simulink library "fzgbib"  (Simulink 4.1.1)
values from neighbouring files (symbols this model uses):
  a_Fzg_max = 2    [PedalInterp_para.m]
  a_Fzg_min = -2    [PedalInterp_para.m]
  gang0 = 1    [PedalInterp_para.m]
  gang_vec = [1 2 3 4]    [PedalInterp_para.m]
  lambda_gang = [1.3 1.25  1.17  1.05]    [PedalInterp_para.m]
  M_Br_max = 4000    [PedalInterp_para.m]
undefined symbols (not defined in the file or in its folder): A, cw, gang, i_d, i_g, m_ab_100pro, m_ab_70pro, m_Fzg, M_mot_max, M_mot_min, n_mot0, n_mot_max, n_mot_min, p_anteil, r_dyn, rho, t_sch, v_bereich, v_Fzg_ms0
libraries: simulink3 x1
(part 2 of 2)

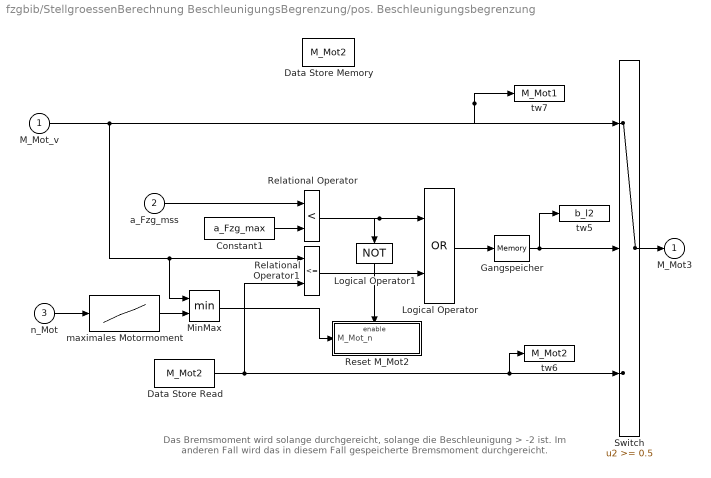
== system fzgbib/StellgroessenBerechnung BeschleunigungsBegrenzung/pos. Beschleunigungsbegrenzung ==
  note: Das Bremsmoment wird solange durchgereicht, solange die Beschleunigung > -2 ist.
      | Im anderen Fall wird das in diesem Fall gespeicherte Bremsmoment durchgereicht.
  M_Mot_v : Inport  Port=1  LatchInput=off
  a_Fzg_mss : Inport  Port=2  LatchInput=off
  "n_Mot " : Inport  Port=3  LatchInput=off
  Constant1 : Constant  Value=a_Fzg_max
  Data Store Memory : DataStoreMemory  DataStoreName=M_Mot2  InitialValue=0
  Data Store Read : DataStoreRead  DataStoreName=M_Mot2  SampleTime=-1
  Gangspeicher : Memory  X0=1  InheritSampleTime=off
      settings: RTWStateStorageClass=Auto
  Logical Operator : Logic  Operator=OR  Inputs=2
  Logical Operator1 : Logic  Orientation=down  Operator=NOT  Inputs=1
  MinMax : MinMax  Function=min  Inputs=2
  Relational Operator : RelationalOperator  Operator=<
  Relational Operator1 : RelationalOperator  Operator=<=
  Reset M_Mot2 : Subsystem  TreatAsAtomicUnit=on
      settings: RTWFcnNameOpts=Auto  RTWFileNameOpts=Auto
  Switch : Switch  Threshold=0.5
  maximales Motormoment : Lookup  InputValues=[0 n_mot_max]  OutputValues=[M_mot_max(1) M_mot_max]
  tw5 : ToWorkspace  VariableName=b_l2  SampleTime=0  SaveFormat=Array
      settings: MaxDataPoints=speicher
  tw6 : ToWorkspace  VariableName=M_Mot2  SampleTime=0  SaveFormat=Array
      settings: MaxDataPoints=speicher
  tw7 : ToWorkspace  VariableName=M_Mot1  SampleTime=0  SaveFormat=Array
      settings: MaxDataPoints=speicher
  M_Mot3 : Outport  Port=1  InitialOutput=0
  wires:
  maximales Motormoment/1 -> MinMax/2
  "n_Mot "/1 -> maximales Motormoment/1
  MinMax/1 -> Reset M_Mot2/1(M_Mot_n)
  a_Fzg_mss/1 -> Relational Operator/1
  Logical Operator1/1 -> Reset M_Mot2/Enable
  Relational Operator/1 -> Logical Operator1/1, Logical Operator/1
  M_Mot_v/1 -> MinMax/1, Relational Operator1/1, tw7/1, Switch/1
  Gangspeicher/1 -> tw5/1, Switch/2
  Logical Operator/1 -> Gangspeicher/1
  Data Store Read/1 -> Relational Operator1/2, tw6/1, Switch/3
  Relational Operator1/1 -> Logical Operator/2
  Constant1/1 -> Relational Operator/2
  Switch/1 -> M_Mot3/1

== system fzgbib/Watchdog 1/error dedected ==
  Enable : EnablePort
  Constant : Constant  Value=1
  max_overshoot_flag [0/1] : Outport  Port=1  InitialOutput=0
  wires:
  Constant/1 -> max_overshoot_flag [0/1]/1

== system fzgbib/Watchdog 1/save actual and reference speed ==
  "actual  speed " : Inport  Port=1  LatchInput=off
  "reference  speed  " : Inport  Port=2  LatchInput=off
  Enable : EnablePort
  actual  speed hold : Outport  Port=1  InitialOutput=0
  reference  speed hold : Outport  Port=2  InitialOutput=0
  wires:
  "reference  speed  "/1 -> reference  speed hold/1
  "actual  speed "/1 -> actual  speed hold/1

== system fzgbib/Watchdog 2/error dedected ==
  Enable : EnablePort
  Constant : Constant  Value=1
  step_response_flag [0/1] : Outport  Port=1  InitialOutput=0
  wires:
  Constant/1 -> step_response_flag [0/1]/1

== system fzgbib/Watchdog 2/save actual time and reference speed ==
  "actual time " : Inport  Port=1  LatchInput=off
  "reference speed  " : Inport  Port=2  LatchInput=off
  Enable : EnablePort
  actual time hold : Outport  Port=1  InitialOutput=0
  reference speed hold : Outport  Port=2  InitialOutput=0
  wires:
  "reference speed  "/1 -> reference speed hold/1
  "actual time "/1 -> actual time hold/1

== system fzgbib/Fahrzeugmodell/Fahrwiderstaende/Schaltdauer ==
  note: Eine Wunschgangaenderung wird registriert und der neue Wunschgang solange im Speicher abgelegt,
      | bis die Schlatung beendet ist.
  note: 14.5.1996 Dieter Hoetzer / letzte aenderung
  Gang_w : Inport  Port=1  LatchInput=off
  Memory1 : Memory  X0=1  InheritSampleTime=off
      settings: RTWStateStorageClass=Auto
  Relational Operator1 : RelationalOperator  Operator=~=
  Schaltdauer : TransportDelay  DelayTime=t_sch  InitialInput=1  BufferSize=1024  PadeOrder=0
  Speicher : Memory  X0=1  InheritSampleTime=off
      settings: RTWStateStorageClass=Auto
  Switch : Switch  Threshold=0.5
  ungleich : RelationalOperator  Operator=~=
  k_l : Outport  Port=1  InitialOutput=0
  wires:
  Switch/1 -> Speicher/1
  Gang_w/1 -> ungleich/1, Switch/1, Memory1/1
  Memory1/1 -> ungleich/2
  ungleich/1 -> Switch/2
  Speicher/1 -> Switch/3, Relational Operator1/1, Schaltdauer/1
  Schaltdauer/1 -> Relational Operator1/2
  Relational Operator1/1 -> k_l/1

== system fzgbib/Fahrzeugmodell/Fahrzeugdynamik/Band-Limited White Noise ==
  Gain : Gain  Gain=[sqrt(Cov)]/[sqrt(Ts)]  Multiplication=Element-wise(K.*u)  SaturateOnIntegerOverflow=on
  White Noise : RandomNumber  Mean=0  Variance=1  Seed=seed  SampleTime=-1
  Zero-Order Hold : ZeroOrderHold  SampleTime=Ts
  Out_1 : Outport  Port=1  InitialOutput=0
  wires:
  Zero-Order Hold/1 -> Gain/1
  Gain/1 -> Out_1/1
  White Noise/1 -> Zero-Order Hold/1

== system fzgbib/Gangberechnung/Hoch-Rueckschaltung Auswahl/Halte Zeit ==
  Clock : Inport  Port=1  LatchInput=off
  Enable : EnablePort
  Write : DataStoreWrite  DataStoreName=time1  SampleTime=-1
  wires:
  Clock/1 -> Write/1

== system fzgbib/GeschwindigkeitsRegelung/Stoergroessenkompensation/Luft- und Rollwiderstand ==
  note: Keine Steigung beruecksichtigt
  v_Fzg : Inport  Port=1  LatchInput=off
  F_L Berechnung : Fcn  Expr=u*rho*A/2*cw
  F_R Berechnung : Fcn  Expr=(u>0.1)*f_r*m_Fzg*g
  Fcn : Fcn  Expr=u*r_dyn
  Product : Product  Inputs=2  Multiplication=Element-wise(.*)  SaturateOnIntegerOverflow=on
  Sum : Sum  Inputs=++  SaturateOnIntegerOverflow=on
  M_G : Outport  Port=1  InitialOutput=0
  wires:
  Fcn/1 -> M_G/1
  Sum/1 -> Fcn/1
  F_L Berechnung/1 -> Sum/1
  F_R Berechnung/1 -> Sum/2
  v_Fzg/1 -> F_R Berechnung/1, Product/1, Product/2
  Product/1 -> F_L Berechnung/1

== system fzgbib/GeschwindigkeitsRegelung/Stoergroessenkompensation/Sollverhalten Fahrzeug mit P-Regler1 ==
  v_soll : Inport  Port=1  LatchInput=off
  v_Fzg : Inport  Port=2  LatchInput=off
  GR_aktiv_l : Inport  Port=3  LatchInput=off
  1/T : Fcn  Expr=1/u
  Grenze3 : Constant  Value=r_dyn*m_Fzg/p_anteil
  Grenze4 : Constant  Value=0.1
  Integrator : Integrator  ExternalReset=none  InitialConditionSource=internal  InitialCondition=v_Fzg_ms0  LimitOutput=off  UpperSaturationLimit=inf  LowerSaturationLimit=-inf  ShowSaturationPort=off  ShowStatePort=off  AbsoluteTolerance=auto
  Product : Product  Inputs=2  Multiplication=Element-wise(.*)  SaturateOnIntegerOverflow=on
  Reglerabweichung : Sum  Inputs=-+  SaturateOnIntegerOverflow=on
  Switch : Switch  Threshold=0.5
  Switch1 : Switch  Threshold=0.5
  v_Fzg1 : Outport  Port=1  InitialOutput=0
  wires:
  Integrator/1 -> v_Fzg1/1, Reglerabweichung/1
  Product/1 -> Integrator/1
  Switch/1 -> 1/T/1
  Reglerabweichung/1 -> Product/1
  1/T/1 -> Product/2
  Grenze4/1 -> Switch/3
  Grenze3/1 -> Switch/1
  Switch1/1 -> Reglerabweichung/2
  v_soll/1 -> Switch1/1
  v_Fzg/1 -> Switch1/3
  GR_aktiv_l/1 -> Switch/2, Switch1/2

== system fzgbib/StellgroessenBerechnung BeschleunigungsBegrenzung/neg. Beschleunigungsbegrenzung/Reset M_Br2 ==
  M_Br_n : Inport  Port=1  LatchInput=off
  a_Fzg_mss : Inport  Port=2  LatchInput=off
  Enable : EnablePort
  Constant1 : Constant  Value=a_Fzg_min
  Constant2 : Constant  Value=10
  Data Store Write : DataStoreWrite  DataStoreName=M_Br2  SampleTime=-1
  Product : Product  Inputs=2  Multiplication=Element-wise(.*)  SaturateOnIntegerOverflow=on
  Sum : Sum  Inputs=++  SaturateOnIntegerOverflow=on
  Sum1 : Sum  Inputs=+-  SaturateOnIntegerOverflow=on
  wires:
  Constant2/1 -> Product/1
  Constant1/1 -> Sum1/2
  a_Fzg_mss/1 -> Sum1/1
  Sum1/1 -> Product/2
  M_Br_n/1 -> Sum/1
  Sum/1 -> Data Store Write/1

== system fzgbib/StellgroessenBerechnung BeschleunigungsBegrenzung/pos. Beschleunigungsbegrenzung/Reset M_Mot2 ==
  M_Mot_n : Inport  Port=1  LatchInput=off
  Enable : EnablePort
  Data Store Write : DataStoreWrite  DataStoreName=M_Mot2  SampleTime=-1
  wires:
  M_Mot_n/1 -> Data Store Write/1
